simulink model "LKAS_AutoSave_DF_20220414_1924_SW62"  (R2018b)
settings: Solver=FixedStepDiscrete  StartTime=0.0  StopTime=10.0  FixedStep=0.01  RelTol=1e-3
model workspace (MAT data in the model file):
  MCOS : class17 (value not decoded)
  MCOS : class17 (value not decoded)
  MCOS : class17 (value not decoded)
  MCOS : class17 (value not decoded)
  MCOS : class17 (value not decoded)
  MCOS : class17 (value not decoded)
  MCOS : class17 (value not decoded)
  MCOS : class17 (value not decoded)
  MCOS : class17 (value not decoded)
  MCOS : class17 (value not decoded)
  MCOS : class17 (value not decoded)
  MCOS : class17 (value not decoded)
  MCOS : class17 (value not decoded)
  MCOS : class17 (value not decoded)
  MCOS : class17 (value not decoded)
  MCOS : class17 (value not decoded)
  MCOS : class17 (value not decoded)
  MCOS : class17 (value not decoded)
  MCOS : class17 (value not decoded)
  MCOS : class17 (value not decoded)
  MCOS : class17 (value not decoded)
  MCOS : class17 (value not decoded)
  MCOS : class17 (value not decoded)
  MCOS : class17 (value not decoded)
  MCOS : class17 (value not decoded)
  MCOS : class17 (value not decoded)
  MCOS : class17 (value not decoded)
  MCOS : class17 (value not decoded)
  MCOS : class17 (value not decoded)
  MCOS : class17 (value not decoded)
  MCOS : class17 (value not decoded)
  MCOS : class17 (value not decoded)
  MCOS : class17 (value not decoded)
  MCOS : class17 (value not decoded)
  MCOS : class17 (value not decoded)
  MCOS : class17 (value not decoded)
  MCOS : class17 (value not decoded)
  MCOS : class17 (value not decoded)
  MCOS : class17 (value not decoded)
  MCOS : class17 (value not decoded)
  MCOS : class17 (value not decoded)
  MCOS : class17 (value not decoded)
  MCOS : class17 (value not decoded)
  MCOS : class17 (value not decoded)
  MCOS : class17 (value not decoded)
  MCOS : class17 (value not decoded)
  MCOS : class17 (value not decoded)
  MCOS : class17 (value not decoded)
  MCOS : class17 (value not decoded)
  MCOS : class17 (value not decoded)
  MCOS : class17 (value not decoded)
  MCOS : class17 (value not decoded)
  MCOS : class17 (value not decoded)
  MCOS : class17 (value not decoded)
  MCOS : class17 (value not decoded)
  MCOS : class17 (value not decoded)
  MCOS : class17 (value not decoded)
  MCOS : class17 (value not decoded)
  MCOS : class17 (value not decoded)
  MCOS : class17 (value not decoded)
  MCOS : class17 (value not decoded)
  MCOS : class17 (value not decoded)
  MCOS : class17 (value not decoded)
  MCOS : class17 (value not decoded)
  MCOS : class17 (value not decoded)
  MCOS : class17 (value not decoded)
  MCOS : class17 (value not decoded)
  MCOS : class17 (value not decoded)
  MCOS : class17 (value not decoded)
  MCOS : class17 (value not decoded)
  MCOS : class17 (value not decoded)
  MCOS : class17 (value not decoded)
  MCOS : class17 (value not decoded)
  MCOS : class17 (value not decoded)
  MCOS : class17 (value not decoded)
  MCOS : class17 (value not decoded)
  MCOS : class17 (value not decoded)
  MCOS : class17 (value not decoded)
  MCOS : class17 (value not decoded)
  MCOS : class17 (value not decoded)
  MCOS : class17 (value not decoded)
  MCOS : class17 (value not decoded)
  MCOS : class17 (value not decoded)
  MCOS : class17 (value not decoded)
  MCOS : class17 (value not decoded)
  MCOS : class17 (value not decoded)
  MCOS : class17 (value not decoded)
  MCOS : class17 (value not decoded)
  MCOS : class17 (value not decoded)
  MCOS : class17 (value not decoded)
  MCOS : class17 (value not decoded)
  MCOS : class17 (value not decoded)
  MCOS : class17 (value not decoded)
  MCOS : class17 (value not decoded)
  MCOS : class17 (value not decoded)
  MCOS : class17 (value not decoded)
  MCOS : class17 (value not decoded)
  MCOS : class17 (value not decoded)
  MCOS : class17 (value not decoded)
  MCOS : class17 (value not decoded)
  MCOS : class17 (value not decoded)
  MCOS : class17 (value not decoded)
  MCOS : class17 (value not decoded)
  MCOS : class17 (value not decoded)
  MCOS : class17 (value not decoded)
  MCOS : class17 (value not decoded)
  MCOS : class17 (value not decoded)
  MCOS : class17 (value not decoded)
  MCOS : class17 (value not decoded)
undefined symbols (not defined in the file): LKA_CarWidth, LKA_SampleTime, LKA_StrRatio_C, LKA_Veh2CamL_C, LKA_Veh2CamW_C, LKA_WhlBaseL_C, LL_CompHdAg_C, LL_CompSWA_C, LL_CrvtPrvwT_C, LL_DesDvt_C, LL_DvtComp_C, LL_DvtPrvwT_C, LL_DvtSpdDet_vDvtSpdMin_C, LL_HandsOff_ExitTime, LL_HandsOff_TextTime, LL_HandsOff_WarnTime, LL_HdAgExT_C, LL_HdAgPrvwT_C, LL_LAccMax_C, LL_LAccRMax_C, LL_LDW_EarliestWarnLine_C, LL_LDW_LatestWarnLine_C, LL_LDWS_SUPPRESS_HEADING, LL_LFClb_TFC_FfCtlRatio_C, LL_LFClb_TFC_KdBalance_C, LL_LFClb_TFC_KdMaxSWA_C, LL_LFClb_TFC_KdV1_C, LL_LFClb_TFC_KdV2_C, LL_LFClb_TFC_KdVehSpdLwr_C, LL_LFClb_TFC_KdVehSpdUpr_C, LL_LFClb_TFC_Ki_C, LL_LFClb_TFC_KiMaxSWA_C, LL_LFClb_TFC_Kp_C, LL_LFClb_TFC_KpKlat_C, LL_LFClb_TFC_KpV1_C, LL_LFClb_TFC_KpV2_C, LL_LFClb_TFC_KpVehSpdLwr_C, LL_LFClb_TFC_KpVehSpdUpr_C, LL_LFClb_TFC_PrvwT_C, LL_LKA_EarliestWarnLine_C, LL_LKA_EnableLine_DvtMax, LL_LKA_EnableLine_DvtMin, LL_LKA_EnableLine_Max, LL_LKA_LatestWarnLine_C, LL_LKAExPrcs_ExitC0Dvt, LL_LKAExPrcs_ExitC0Swt, LL_LKAExPrcs_tiExitDelayTime3, LL_LKAExPrcs_tiExitTime1, LL_LKAExPrcs_tiExitTime2, LL_LKAExPrcs_tiExitTime3, LL_LKAS_OUT_OF_CONTROL_LAT_VEL, LL_LKAS_OUT_OF_CONTROL_TTLC, LL_LKASWASyn_M0, LL_LKASWASyn_M1, LL_LKASWASyn_M2, LL_LKASWASyn_M3D, LL_LKASWASyn_M3K_DT, LL_LKASWASyn_M3K_MSD, LL_LKASWASyn_M4K, LL_LKASWASyn_SWAaddMax ... (+50)
libraries: simulink x234, canmsglib x6, dspstat3 x3, simulink_extras x1
(part 4 of 17)

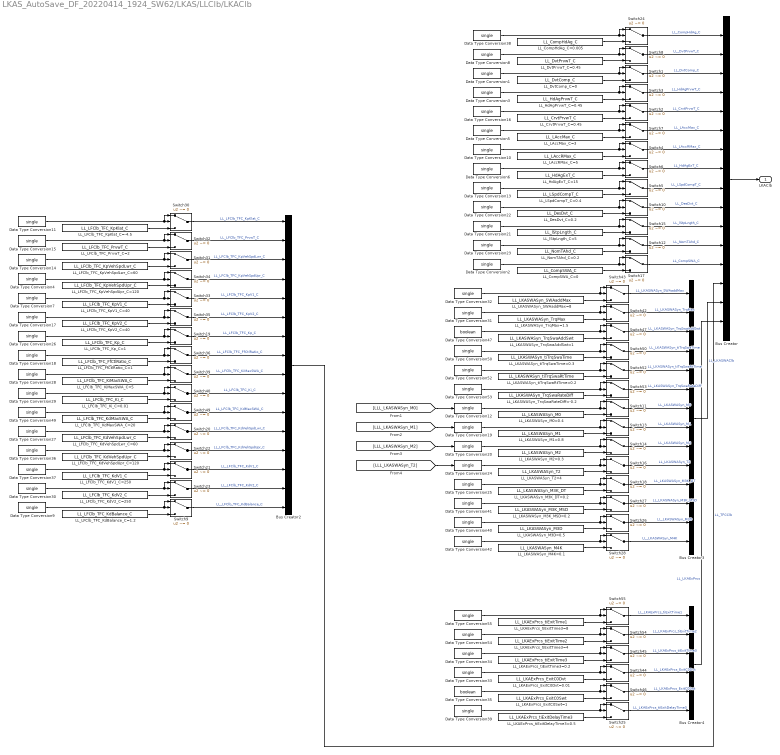
== system LKAS_AutoSave_DF_20220414_1924_SW62/LKAS/LLClb/LKAClb ==
  Bus Creator : BusCreator  Inputs=16
  Bus Creator2 : BusCreator  Inputs=16
  Bus Creator3 : BusCreator  Inputs=14
  Bus Creator4 : BusCreator  Inputs=6
  Data Type Conversion{1..34,36..42,49..50,52..55} (47 alike) : DataTypeConversion  OutDataTypeStr=single
  Data Type Conversion35 : DataTypeConversion  OutDataTypeStr=boolean
  Data Type Conversion47 : DataTypeConversion  OutDataTypeStr=boolean
  LL_CompHdAg_C=0.005 : Constant  Value=LL_CompHdAg_C  OutDataTypeStr=single
  LL_CompSWA_C=0 : Constant  Value=LL_CompSWA_C  OutDataTypeStr=single
  LL_CrvtPrvwT_C=0.45 : Constant  Value=LL_CrvtPrvwT_C  OutDataTypeStr=single
  LL_DesDvt_C=0.2 : Constant  Value=LL_DesDvt_C  OutDataTypeStr=single
  LL_DvtComp_C=0 : Constant  Value=LL_DvtComp_C  OutDataTypeStr=single
  LL_DvtPrvwT_C=0.45 : Constant  Value=LL_DvtPrvwT_C  OutDataTypeStr=single
  LL_HdAgExT_C=15 : Constant  Value=LL_HdAgExT_C  OutDataTypeStr=single
  LL_HdAgPrvwT_C=0.45 : Constant  Value=LL_HdAgPrvwT_C  OutDataTypeStr=single
  LL_LAccMax_C=3 : Constant  Value=LL_LAccMax_C  OutDataTypeStr=single
  LL_LAccRMax_C=5 : Constant  Value=LL_LAccRMax_C  OutDataTypeStr=single
  LL_LFClb_TFC_FfCtlRatio_C=1 : Constant  Value=LL_LFClb_TFC_FfCtlRatio_C  OutDataTypeStr=single
  LL_LFClb_TFC_KdBalance_C=1.2 : Constant  Value=LL_LFClb_TFC_KdBalance_C  OutDataTypeStr=single
  LL_LFClb_TFC_KdMaxSWA_C=20 : Constant  Value=LL_LFClb_TFC_KdMaxSWA_C  OutDataTypeStr=single
  LL_LFClb_TFC_KdV1_C=250 : Constant  Value=LL_LFClb_TFC_KdV1_C  OutDataTypeStr=single
  LL_LFClb_TFC_KdV2_C=250 : Constant  Value=LL_LFClb_TFC_KdV2_C  OutDataTypeStr=single
  LL_LFClb_TFC_KdVehSpdLwr_C=60 : Constant  Value=LL_LFClb_TFC_KdVehSpdLwr_C  OutDataTypeStr=single
  LL_LFClb_TFC_KdVehSpdUpr_C=120 : Constant  Value=LL_LFClb_TFC_KdVehSpdUpr_C  OutDataTypeStr=single
  LL_LFClb_TFC_KiMaxSWA_C=5 : Constant  Value=LL_LFClb_TFC_KiMaxSWA_C  OutDataTypeStr=single
  LL_LFClb_TFC_Ki_C=0.01 : Constant  Value=LL_LFClb_TFC_Ki_C  OutDataTypeStr=single
  LL_LFClb_TFC_KpKlat_C=-4.5 : Constant  Value=LL_LFClb_TFC_KpKlat_C  OutDataTypeStr=single
  LL_LFClb_TFC_KpV1_C=40 : Constant  Value=LL_LFClb_TFC_KpV1_C  OutDataTypeStr=single
  LL_LFClb_TFC_KpV2_C=40 : Constant  Value=LL_LFClb_TFC_KpV2_C  OutDataTypeStr=single
  LL_LFClb_TFC_KpVehSpdLwr_C=60 : Constant  Value=LL_LFClb_TFC_KpVehSpdLwr_C  OutDataTypeStr=single
  LL_LFClb_TFC_KpVehSpdUpr_C=120 : Constant  Value=LL_LFClb_TFC_KpVehSpdUpr_C  OutDataTypeStr=single
  LL_LFClb_TFC_Kp_C=1 : Constant  Value=LL_LFClb_TFC_Kp_C  OutDataTypeStr=single
  LL_LFClb_TFC_PrvwT_C=2 : Constant  Value=LL_LFClb_TFC_PrvwT_C  OutDataTypeStr=single
  LL_LKAExPrcs_ExitC0Dvt=0.01 : Constant  Value=LL_LKAExPrcs_ExitC0Dvt  OutDataTypeStr=single
  LL_LKAExPrcs_ExitC0Swt=1 : Constant  Value=LL_LKAExPrcs_ExitC0Swt  OutDataTypeStr=boolean
  LL_LKAExPrcs_tiExitDelayTime3=0.5 : Constant  Value=LL_LKAExPrcs_tiExitDelayTime3  OutDataTypeStr=single
  LL_LKAExPrcs_tiExitTime3=0.2 : Constant  Value=LL_LKAExPrcs_tiExitTime3  OutDataTypeStr=single
  LL_LKAExPrcs_tiExitTime3=4 : Constant  Value=LL_LKAExPrcs_tiExitTime2  OutDataTypeStr=single
  LL_LKAExPrcs_tiExitTime3=8 : Constant  Value=LL_LKAExPrcs_tiExitTime1  OutDataTypeStr=single
  LL_LKASWASyn_M0=0.4 : Constant  Value=LL_LKASWASyn_M0  OutDataTypeStr=single
  LL_LKASWASyn_M1=0.8 : Constant  Value=LL_LKASWASyn_M1  OutDataTypeStr=single
  LL_LKASWASyn_M2=0.3 : Constant  Value=LL_LKASWASyn_M2  OutDataTypeStr=single
  LL_LKASWASyn_M3D=0.5 : Constant  Value=LL_LKASWASyn_M3D  OutDataTypeStr=single
  LL_LKASWASyn_M3K_DT=0.2 : Constant  Value=LL_LKASWASyn_M3K_DT  OutDataTypeStr=single
  LL_LKASWASyn_M3K_MSD=0.2 : Constant  Value=LL_LKASWASyn_M3K_MSD  OutDataTypeStr=single
  LL_LKASWASyn_M4K=0.1 : Constant  Value=LL_LKASWASyn_M4K  OutDataTypeStr=single
  LL_LKASWASyn_SWAaddMax=8 : Constant  Value=LL_LKASWASyn_SWAaddMax  OutDataTypeStr=single
  LL_LKASWASyn_T2=4 : Constant  Value=LL_LKASWASyn_T2  OutDataTypeStr=single
  LL_LKASWASyn_TrqMax=1.5 : Constant  Value=LL_LKASWASyn_TrqMax  OutDataTypeStr=single
  LL_LKASWASyn_TrqSwaAddSwt=1 : Constant  Value=LL_LKASWASyn_TrqSwaAddSwt  OutDataTypeStr=boolean
  LL_LKASWASyn_TrqSwaRateDiff=-0.2 : Constant  Value=LL_LKASWASyn_TrqSwaRateDiff  OutDataTypeStr=single
  LL_LKASWASyn_tiTrqSwaRtTime=0.2 : Constant  Value=LL_LKASWASyn_tiTrqSwaRtTime  OutDataTypeStr=single
  LL_LKASWASyn_tiTrqSwaTime=0.3 : Constant  Value=LL_LKASWASyn_tiTrqSwaTime  OutDataTypeStr=single
  LL_LSpdCompT_C=0.4 : Constant  Value=LL_LSpdCompT_C  OutDataTypeStr=single
  LL_NomTAhd_C=0.2 : Constant  Value=LL_NomTAhd_C  OutDataTypeStr=single
  LL_lStpLngth_C=5 : Constant  Value=LL_lStpLngth_C  OutDataTypeStr=single
  Switch{1..28,30..36,39..40,42..45,49..50,52..55} (47 alike) : Switch  Criteria=u2 ~= 0  OutDataTypeStr=single
  Switch46 : Switch  Criteria=u2 ~= 0  OutDataTypeStr=boolean
  Switch47 : Switch  Criteria=u2 ~= 0  OutDataTypeStr=boolean
  LKAClb : Outport
  wires:
  Data Type Conversion42/1 -> Switch28/2, Switch28/1
  LL_LKASWASyn_M4K=0.1/1 -> Switch28/3
  Switch28/1 -> Bus Creator3/14  "LL_LKASWASyn_M4K"
  Switch27/1 -> Bus Creator3/12  "LL_LKASWASyn_M3K_MSD"
  LL_LKASWASyn_M3K_MSD=0.2/1 -> Switch27/3
  Data Type Conversion41/1 -> Switch27/1, Switch27/2
  Switch26/1 -> Bus Creator3/13  "LL_LKASWASyn_M3D"
  LL_LKASWASyn_M3D=0.5/1 -> Switch26/3
  Data Type Conversion40/1 -> Switch26/1, Switch26/2
  Data Type Conversion39/1 -> Switch25/2, Switch25/1
  Switch25/1 -> Bus Creator4/6  "LL_LKAExPrcs_tiExitDelayTime3"
  LL_LKAExPrcs_tiExitDelayTime3=0.5/1 -> Switch25/3
  LL_CompHdAg_C=0.005/1 -> Switch24/3
  Data Type Conversion38/1 -> Switch24/1, Switch24/2
  Switch24/1 -> Bus Creator/1  "LL_CompHdAg_C"
  Data Type Conversion37/1 -> Switch21/2, Switch21/1
  LL_LFClb_TFC_KdV2_C=250/1 -> Switch23/3
  Switch23/1 -> Bus Creator2/15  "LL_LFClb_TFC_KdV2_C"
  LL_LFClb_TFC_KdVehSpdUpr_C=120/1 -> Switch22/3
  Switch20/1 -> Bus Creator2/12  "LL_LFClb_TFC_KdVehSpdLwr_C"
  Switch22/1 -> Bus Creator2/13  "LL_LFClb_TFC_KdVehSpdUpr_C"
  Data Type Conversion27/1 -> Switch20/2, Switch20/1
  Data Type Conversion36/1 -> Switch22/2, Switch22/1
  LL_LFClb_TFC_KdV1_C=250/1 -> Switch21/3
  LL_LFClb_TFC_KdVehSpdLwr_C=60/1 -> Switch20/3
  Switch21/1 -> Bus Creator2/14  "LL_LFClb_TFC_KdV1_C"
  Data Type Conversion30/1 -> Switch23/2, Switch23/1
  LL_LFClb_TFC_Kp_C=1/1 -> Switch19/3
  Switch19/1 -> Bus Creator2/7  "LL_LFClb_TFC_Kp_C"
  Data Type Conversion26/1 -> Switch19/2, Switch19/1
  Bus Creator/1 -> LKAClb/1
  Switch8/1 -> Bus Creator/2  "LL_DvtPrvwT_C"
  Switch1/1 -> Bus Creator/3  "LL_DvtComp_C"
  Switch3/1 -> Bus Creator/4  "LL_HdAgPrvwT_C"
  Switch17/1 -> Bus Creator/13  "LL_CompSWA_C"
  Switch6/1 -> Bus Creator/8  "LL_HdAgExT_C"
  Switch7/1 -> Bus Creator/6  "LL_LAccMax_C"
  Switch4/1 -> Bus Creator/7  "LL_LAccRMax_C"
  Switch5/1 -> Bus Creator/9  "LL_LSpdCompT_C"
  Switch2/1 -> Bus Creator/5  "LL_CrvtPrvwT_C"
  Switch15/1 -> Bus Creator/11  "LL_lStpLngth_C"
  Switch10/1 -> Bus Creator/10  "LL_DesDvt_C"
  Switch12/1 -> Bus Creator/12  "LL_NomTAhd_C"
  LL_DvtPrvwT_C=0.45/1 -> Switch8/3
  Data Type Conversion8/1 -> Switch8/1, Switch8/2
  Data Type Conversion1/1 -> Switch1/2, Switch1/1
  LL_DvtComp_C=0/1 -> Switch1/3
  LL_CrvtPrvwT_C=0.45/1 -> Switch2/3
  Data Type Conversion16/1 -> Switch2/2, Switch2/1
  Data Type Conversion3/1 -> Switch3/2, Switch3/1
  LL_HdAgPrvwT_C=0.45/1 -> Switch3/3
  LL_HdAgExT_C=15/1 -> Switch6/3
  Data Type Conversion6/1 -> Switch6/2, Switch6/1
  Data Type Conversion13/1 -> Switch5/2, Switch5/1
  LL_LSpdCompT_C=0.4/1 -> Switch5/3
  LL_LAccRMax_C=5/1 -> Switch4/3
  Data Type Conversion10/1 -> Switch4/1, Switch4/2
  Data Type Conversion5/1 -> Switch7/2, Switch7/1
  LL_LAccMax_C=3/1 -> Switch7/3
  Data Type Conversion21/1 -> Switch15/2, Switch15/1
  Data Type Conversion23/1 -> Switch12/2, Switch12/1
  Data Type Conversion22/1 -> Switch10/2, Switch10/1
  Data Type Conversion2/1 -> Switch17/2, Switch17/1
  LL_DesDvt_C=0.2/1 -> Switch10/3
  LL_lStpLngth_C=5/1 -> Switch15/3
  LL_NomTAhd_C=0.2/1 -> Switch12/3
  LL_CompSWA_C=0/1 -> Switch17/3
  Bus Creator2/1 -> Bus Creator/14  "LL_TFCClb"
  Switch35/1 -> Bus Creator2/6  "LL_LFClb_TFC_KpV2_C"
  Switch30/1 -> Bus Creator2/1  "LL_LFClb_TFC_KpKlat_C"
  Switch31/1 -> Bus Creator2/3  "LL_LFClb_TFC_KpVehSpdLwr_C"
  Switch34/1 -> Bus Creator2/4  "LL_LFClb_TFC_KpVehSpdUpr_C"
  Switch33/1 -> Bus Creator2/5  "LL_LFClb_TFC_KpV1_C"
  Switch32/1 -> Bus Creator2/2  "LL_LFClb_TFC_PrvwT_C"
  LL_LFClb_TFC_KpV1_C=40/1 -> Switch33/3
  LL_LFClb_TFC_KpVehSpdLwr_C=60/1 -> Switch31/3
  LL_LFClb_TFC_PrvwT_C=2/1 -> Switch32/3
  Data Type Conversion11/1 -> Switch30/2, Switch30/1
  Data Type Conversion7/1 -> Switch33/2, Switch33/1
  Data Type Conversion4/1 -> Switch34/2, Switch34/1
  Data Type Conversion15/1 -> Switch32/2, Switch32/1
  Data Type Conversion17/1 -> Switch35/2, Switch35/1
  LL_LFClb_TFC_KpV2_C=40/1 -> Switch35/3
  Data Type Conversion14/1 -> Switch31/2, Switch31/1
  LL_LFClb_TFC_KpVehSpdUpr_C=120/1 -> Switch34/3
  LL_LFClb_TFC_KpKlat_C=-4.5/1 -> Switch30/3
  LL_LFClb_TFC_FfCtlRatio_C=1/1 -> Switch36/3
  Data Type Conversion18/1 -> Switch36/1, Switch36/2
  Switch36/1 -> Bus Creator2/8  "LL_LFClb_TFC_FfCtlRatio_C"
  Switch40/1 -> Bus Creator2/10  "LL_LFClb_TFC_Ki_C"
  Switch39/1 -> Bus Creator2/9  "LL_LFClb_TFC_KiMaxSWA_C"
  LL_LFClb_TFC_KiMaxSWA_C=5/1 -> Switch39/3
  Data Type Conversion28/1 -> Switch39/1, Switch39/2
  LL_LFClb_TFC_Ki_C=0.01/1 -> Switch40/3
  Data Type Conversion29/1 -> Switch40/1, Switch40/2
  Data Type Conversion31/1 -> Switch42/2, Switch42/1
  LL_LKASWASyn_TrqMax=1.5/1 -> Switch42/3
  LL_LKASWASyn_SWAaddMax=8/1 -> Switch43/3
  Data Type Conversion32/1 -> Switch43/1, Switch43/2
  Switch43/1 -> Bus Creator3/1  "LL_LKASWASyn_SWAaddMax"
  Switch42/1 -> Bus Creator3/2  "LL_LKASWASyn_TrqMax"
  Bus Creator3/1 -> Bus Creator/15  "LL_LKASWAClb"
  Switch44/1 -> Bus Creator4/4  "LL_LKAExPrcs_ExitC0Dvt"
  Switch45/1 -> Bus Creator4/3  "LL_LKAExPrcs_tiExitTime3"
  Data Type Conversion34/1 -> Switch45/2, Switch45/1
  LL_LKAExPrcs_tiExitTime3=0.2/1 -> Switch45/3
  LL_LKAExPrcs_ExitC0Dvt=0.01/1 -> Switch44/3
  Data Type Conversion33/1 -> Switch44/1, Switch44/2
  Bus Creator4/1 -> Bus Creator/16  "LL_LKAExPrcs"
  Data Type Conversion35/1 -> Switch46/2, Switch46/1
  LL_LKAExPrcs_ExitC0Swt=1/1 -> Switch46/3
  Switch46/1 -> Bus Creator4/5  "LL_LKAExPrcs_ExitC0Swt"
  Switch47/1 -> Bus Creator3/3  "LL_LKASWASyn_TrqSwaAddSwt"
  LL_LKASWASyn_TrqSwaAddSwt=1/1 -> Switch47/3
  Data Type Conversion47/1 -> Switch47/1, Switch47/2
  Switch49/1 -> Bus Creator2/11  "LL_LFClb_TFC_KdMaxSWA_C"
  LL_LFClb_TFC_KdMaxSWA_C=20/1 -> Switch49/3
  Data Type Conversion49/1 -> Switch49/1, Switch49/2
  Data Type Conversion50/1 -> Switch50/2, Switch50/1
  LL_LKASWASyn_tiTrqSwaTime=0.3/1 -> Switch50/3
  Switch50/1 -> Bus Creator3/4  "LL_LKASWASyn_tiTrqSwaTime"
  Switch52/1 -> Bus Creator3/5  "LL_LKASWASyn_tiTrqSwaRtTime"
  LL_LKASWASyn_tiTrqSwaRtTime=0.2/1 -> Switch52/3
  Data Type Conversion52/1 -> Switch52/1, Switch52/2
  Data Type Conversion53/1 -> Switch53/2, Switch53/1
  LL_LKASWASyn_TrqSwaRateDiff=-0.2/1 -> Switch53/3
  Switch53/1 -> Bus Creator3/6  "LL_LKASWASyn_TrqSwaRateDiff"
  LL_LKAExPrcs_tiExitTime3=4/1 -> Switch54/3
  Data Type Conversion54/1 -> Switch54/1, Switch54/2
  Switch54/1 -> Bus Creator4/2  "LL_LKAExPrcs_tiExitTime2"
  Switch55/1 -> Bus Creator4/1  "LL_LKAExPrcs_tiExitTime1"
  Data Type Conversion55/1 -> Switch55/2, Switch55/1
  LL_LKAExPrcs_tiExitTime3=8/1 -> Switch55/3
  Switch9/1 -> Bus Creator2/16  "LL_LFClb_TFC_KdBalance_C"
  LL_LFClb_TFC_KdBalance_C=1.2/1 -> Switch9/3
  Data Type Conversion9/1 -> Switch9/1, Switch9/2
  [LLL_LKASWASyn_T2] -> Data Type Conversion24/1
  Switch16/1 -> Bus Creator3/10  "LL_LKASWASyn_T2"
  LL_LKASWASyn_T2=4/1 -> Switch16/3
  Data Type Conversion24/1 -> Switch16/1, Switch16/2
  Data Type Conversion20/1 -> Switch14/2, Switch14/1
  LL_LKASWASyn_M2=0.3/1 -> Switch14/3
  Switch14/1 -> Bus Creator3/9  "LL_LKASWASyn_M2"
  [LLL_LKASWASyn_M2] -> Data Type Conversion20/1
  [LLL_LKASWASyn_M1] -> Data Type Conversion19/1
  Switch13/1 -> Bus Creator3/8  "LL_LKASWASyn_M1"
  LL_LKASWASyn_M1=0.8/1 -> Switch13/3
  Data Type Conversion19/1 -> Switch13/1, Switch13/2
  Data Type Conversion12/1 -> Switch11/2, Switch11/1
  LL_LKASWASyn_M0=0.4/1 -> Switch11/3
  Switch11/1 -> Bus Creator3/7  "LL_LKASWASyn_M0"
  [LLL_LKASWASyn_M0] -> Data Type Conversion12/1
  Data Type Conversion25/1 -> Switch18/2, Switch18/1
  LL_LKASWASyn_M3K_DT=0.2/1 -> Switch18/3
  Switch18/1 -> Bus Creator3/11  "LL_LKASWASyn_M3K_DT"

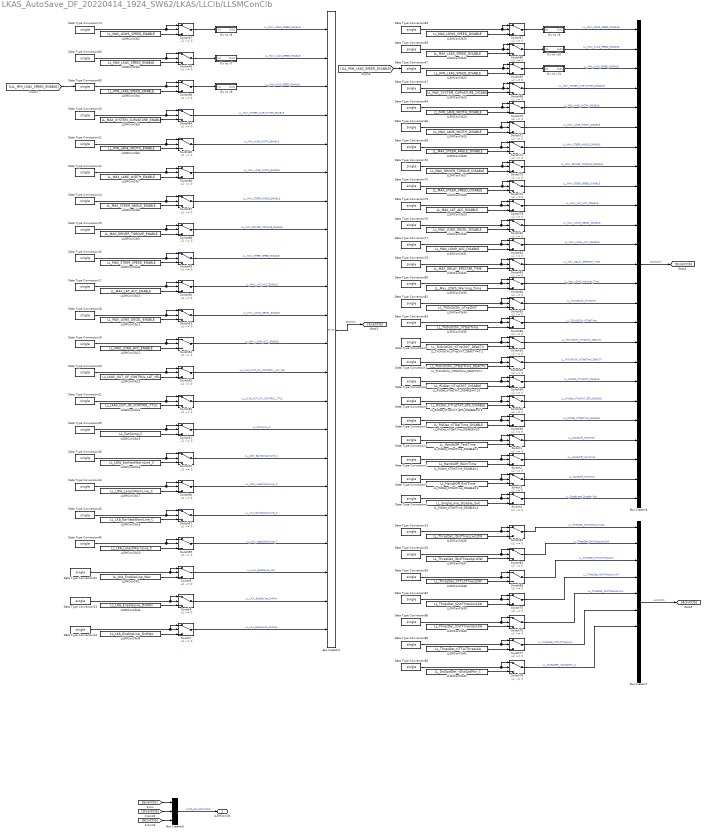
== system LKAS_AutoSave_DF_20220414_1924_SW62/LKAS/LLClb/LLSMConClb ==
  Bus Creator4 : BusCreator  Inputs=22
  Bus Creator5 : BusCreator  Inputs=3
  Bus Creator6 : BusCreator  Inputs=25
  Bus Creator7 : BusCreator  Inputs=10
  Data Type Conversion{1..26,36,44..47,58,64..70,72,74..78,80,82..89} (54 alike) : DataTypeConversion  OutDataTypeStr=single
  ICv to v10 : Subsystem
  ICv to v11 : Subsystem
  ICv to v6 : Subsystem  Description=|
      | 仪表车速转换
      | 仪表车速 = 实际车速 * 1.02 + 2.5
      settings: AttributesFormatString=%<Description>
  ICv to v7 : Subsystem
  ICv to v8 : Subsystem
  ICv to v9 : Subsystem
  LLSMConClb1 : Constant  Description=LKA功能的偏移量使能上限  Value=LL_LKA_EnableLine_Max  OutDataTypeStr=single
      settings: AttributesFormatString=|
      | %<Value>  = 0.4
      | %<Description>
  LLSMConClb10 : Constant  Description=侧向加速度使能上限  Value=LL_MAX_LAT_ACC_ENABLE  OutDataTypeStr=single
      settings: AttributesFormatString=|
      | %<Value>  = 3
      | %<Description>
  LLSMConClb11 : Constant  Description=纵向减速度使能上限  Value=LL_MAX_LONG_DECEL_ENABLE  OutDataTypeStr=single
      settings: AttributesFormatString=|
      | %<Value>  = 2
      | %<Description>
  LLSMConClb12 : Constant  Description=纵向加速度使能上限  Value=LL_MAX_LONG_ACC_ENABLE  OutDataTypeStr=single
      settings: AttributesFormatString=|
      | %<Value>  = 3
      | %<Description>
  LLSMConClb13 : Constant  Description=LKA功能的侧向偏出速度阈值  Value=LL_LKAS_OUT_OF_CONTROL_LAT_VEL  OutDataTypeStr=single
      settings: AttributesFormatString=|
      | %<Value>  = 1.5
      | %<Description>
  LLSMConClb14 : Constant  Description=LKA功能的超过最迟干预线持续时间阈值  Value=LL_LKAS_OUT_OF_CONTROL_TTLC  OutDataTypeStr=single
      settings: AttributesFormatString=|
      | %<Value>  = 0.3
      | %<Description>
  LLSMConClb15 : Constant  Description=偏移量补偿  Value=LL_DvtComp_C  OutDataTypeStr=single
      settings: AttributesFormatString=|
      | %<Value>  = 0
      | %<Description>
  LLSMConClb16 : Constant  Description=LDW功能的最早预警线  Value=LL_LDW_EarliestWarnLine_C  OutDataTypeStr=single
      settings: AttributesFormatString=|
      | %<Value>  = 0.3
      | %<Description>
  LLSMConClb17 : Constant  Description=LDW功能的最迟预警线  Value=LL_LDW_LatestWarnLine_C  OutDataTypeStr=single
      settings: AttributesFormatString=|
      | %<Value>  = -0.4
      | %<Description>
  LLSMConClb18 : Constant  Description=LKA功能的最早预警线  Value=LL_LKA_EarliestWarnLine_C  OutDataTypeStr=single
      settings: AttributesFormatString=|
      | %<Value>  = 0.3
      | %<Description>
  LLSMConClb19 : Constant  Description=LKA功能的最迟预警线  Value=LL_LKA_LatestWarnLine_C  OutDataTypeStr=single
      settings: AttributesFormatString=|
      | %<Value>  = -0.5
      | %<Description>
  LLSMConClb2 : Constant  Description=LDW功能的车速使能上限  Value=LL_MAX_LDWS_SPEED_ENABLE  OutDataTypeStr=single
      settings: AttributesFormatString=|
      | %<Value>  = 140
      | %<Description>
  LLSMConClb20 : Constant  Description=LDW功能的车速失效上限  Value=LL_MAX_LDWS_SPEED_DISABLE  OutDataTypeStr=single
      settings: AttributesFormatString=|
      | %<Value>  = 150
      | %<Description>
  LLSMConClb21 : Constant  Description=LKA功能的车速失效上限  Value=LL_MAX_LKAS_SPEED_DISABLE  OutDataTypeStr=single
      settings: AttributesFormatString=|
      | %<Value>  = 150
      | %<Description>
  LLSMConClb22 : Constant  Description=LKA功能的车速失效下限  Value=LL_MIN_LKAS_SPEED_DISABLE  OutDataTypeStr=single
      settings: AttributesFormatString=|
      | %<Value>  = 55
      | %<Description>
  LLSMConClb23 : Constant  Description=曲率失效上限  Value=LL_MAX_SYSTEM_CURVATURE_DISABLE  OutDataTypeStr=single
      settings: AttributesFormatString=|
      | %<Value>  = 0.0055
      | %<Description>
  LLSMConClb24 : Constant  Description=车道线宽度失效下限  Value=LL_MIN_LANE_WIDTH_DISABLE  OutDataTypeStr=single
      settings: AttributesFormatString=|
      | %<Value>  = 2.4
      | %<Description>
  LLSMConClb25 : Constant  Description=车道线宽度失效上限  Value=LL_MAX_LANE_WIDTH_DISABLE  OutDataTypeStr=single
      settings: AttributesFormatString=|
      | %<Value>  = 5.5
      | %<Description>
  LLSMConClb26 : Constant  Description=方向盘转角退出上限  Value=LL_MAX_STEER_ANGLE_DISABLE  OutDataTypeStr=single
      settings: AttributesFormatString=|
      | %<Value>  = 70
      | %<Description>
  LLSMConClb27 : Constant  Description=驾驶员转矩失效上限  Value=LL_MAX_DRIVER_TORQUE_DISABLE  OutDataTypeStr=single
      settings: AttributesFormatString=|
      | %<Value>  = 2.25
      | %<Description>
  LLSMConClb28 : Constant  Description=方向盘转速失效上限  Value=LL_MAX_STEER_SPEED_DISABLE  OutDataTypeStr=single
      settings: AttributesFormatString=|
      | %<Value>  = 5000
      | %<Description>
  LLSMConClb29 : Constant  Description=侧向加速度失效上限  Value=LL_MAX_LAT_ACC_DISABLE  OutDataTypeStr=single
      settings: AttributesFormatString=|
      | %<Value>  = 3.5
      | %<Description>
  LLSMConClb3 : Constant  Description=LKA功能的车速使能上限  Value=LL_MAX_LKAS_SPEED_ENABLE  OutDataTypeStr=single
      settings: AttributesFormatString=|
      | %<Value>  = 140
      | %<Description>
  LLSMConClb30 : Constant  Description=纵向减速度失效上限  Value=LL_MAX_LONG_DECEL_DISABLE  OutDataTypeStr=single
      settings: AttributesFormatString=|
      | %<Value>  = 2.5
      | %<Description>
  LLSMConClb31 : Constant  Description=纵向加速度失效上限  Value=LL_MAX_LONG_ACC_DISABLE  OutDataTypeStr=single
      settings: AttributesFormatString=|
      | %<Value>  = 3.5
      | %<Description>
  LLSMConClb32 : Constant  Description=LKA功能的EPS延迟进入等待的时间上限  Value=LL_MAX_DELAY_EPSSTAR_TIME  OutDataTypeStr=single
      settings: AttributesFormatString=|
      | %<Value>  = 0.5
      | %<Description>
  LLSMConClb33 : Constant  Description=LDW功能的连续报警时间上限  Value=LL_Max_LDWS_Warning_Time  OutDataTypeStr=single
      settings: AttributesFormatString=|
      | %<Value>  = 5
      | %<Description>
  LLSMConClb34 : Constant  Description=驾驶员接管时间阈值  Value=LL_TkOvStChk_tiTrqChkT  OutDataTypeStr=single
      settings: AttributesFormatString=|
      | %<Value>  = 0.1
      | %<Description>
  LLSMConClb35 : Constant  Description=距离上次驾驶员接管时间间隔  Value=LL_TkOvStChk_tiTDelTime  OutDataTypeStr=single
      settings: AttributesFormatString=|
      | %<Value>  = 2
      | %<Description>
  LLSMConClb36 : Constant  Description=LDW功能的偏移量激活下限  Value=LL_ThresDet_lDvtThresLwrLDW  OutDataTypeStr=single
      settings: AttributesFormatString=|
      | %<Value>  = 0.15
      | %<Description>
  LLSMConClb37 : Constant  Description=LDW功能的偏移量激活上限  Value=LL_ThresDet_lDvtThresUprLDW  OutDataTypeStr=single
      settings: AttributesFormatString=|
      | %<Value>  = 0.3
      | %<Description>
  LLSMConClb38 : Constant  Description=LDW功能的跨道时间激活阈值  Value=LL_ThresDet_tiTTLCThresLDW  OutDataTypeStr=single
      settings: AttributesFormatString=|
      | %<Value>  = 0.75
      | %<Description>
  LLSMConClb39 : Constant  Description=LKA功能的偏移量激活下限  Value=LL_ThresDet_lDvtThresLwrLKA  OutDataTypeStr=single
      settings: AttributesFormatString=|
      | %<Value>  = 0.3
      | %<Description>
  LLSMConClb4 : Constant  Description=LKA功能的车速使能下限  Value=LL_MIN_LKAS_SPEED_ENABLE  OutDataTypeStr=single
      settings: AttributesFormatString=|
      | %<Value>  = 60
      | %<Description>
  LLSMConClb40 : Constant  Description=LKA功能的偏移量激活上限  Value=LL_ThresDet_lDvtThresUprLKA  OutDataTypeStr=single
      settings: AttributesFormatString=|
      | %<Value>  = 0.6
      | %<Description>
  LLSMConClb41 : Constant  Description=LKA功能的跨道时间激活阈值  Value=LL_ThresDet_tiTTLCThresLKA  OutDataTypeStr=single
      settings: AttributesFormatString=|
      | %<Value>  = 1.5
      | %<Description>
  LLSMConClb42 : Constant  Description=偏出侧向速度最小值  Value=LL_DvtSpdDet_vDvtSpdMin_C  OutDataTypeStr=single
      settings: AttributesFormatString=|
      | %<Value>  = 0
      | %<Description>
  LLSMConClb43 : Constant  Description=方向盘转速使能上限  Value=LL_MAX_STEER_SPEED_ENABLE  OutDataTypeStr=single
      settings: AttributesFormatString=|
      | %<Value>  = 5000
      | %<Description>
  LLSMConClb44 : Constant  Description=LKA功能的使能最小车道宽度计算因子  Value=LL_LKA_EnableLine_DvtMin  OutDataTypeStr=single
      settings: AttributesFormatString=|
      | %<Value>  = 0.2
      | %<Description>
  LLSMConClb45 : Constant  Description=LKA功能的使能最大车道宽度计算因子  Value=LL_LKA_EnableLine_DvtMax  OutDataTypeStr=single
      settings: AttributesFormatString=|
      | %<Value>  = 1.2
      | %<Description>
  LLSMConClb5 : Constant  Description=曲率使能上限  Value=LL_MAX_SYSTEM_CURVATURE_ENABLE  OutDataTypeStr=single
      settings: AttributesFormatString=|
      | %<Value>  = 0.0045
      | %<Description>
  LLSMConClb6 : Constant  Description=车道线宽度使能下限  Value=LL_MIN_LANE_WIDTH_ENABLE  OutDataTypeStr=single
      settings: AttributesFormatString=|
      | %<Value>  = 2.5
      | %<Description>
  LLSMConClb7 : Constant  Description=车道线宽度使能上限  Value=LL_MAX_LANE_WIDTH_ENABLE  OutDataTypeStr=single
      settings: AttributesFormatString=|
      | %<Value>  = 5.4
      | %<Description>
  LLSMConClb8 : Constant  Description=方向盘转角使能上限  Value=LL_MAX_STEER_ANGLE_ENABLE  OutDataTypeStr=single
      settings: AttributesFormatString=|
      | %<Value>  = 60
      | %<Description>
  LLSMConClb9 : Constant  Description=驾驶员扭矩使能上限  Value=LL_MAX_DRIVER_TORQUE_ENABLE  OutDataTypeStr=single
      settings: AttributesFormatString=|
      | %<Value>  = 3
      | %<Description>
  LL_RlsDet_tiTDelTime_DISABLE=1 : Constant  Description=驾驶员脱手开始到功能发出动画提醒的时间  Value=LL_HandsOff_TextTime  OutDataTypeStr=single
      settings: AttributesFormatString=|
      | %<Value>  = 10
      | %<Description>
  LL_RlsDet_tiTDelTime_DISABLE=2 : Constant  Description=驾驶员脱手开始到发出声音报警的时间  Value=LL_HandsOff_WarnTime  OutDataTypeStr=single
      settings: AttributesFormatString=|
      | %<Value>  = 15
      | %<Description>
  LL_RlsDet_tiTDelTime_DISABLE=20 : Constant  Description=反使能距离上次驾驶员脱手时间间隔  Value=LL_RlsDet_tiTDelTime_DISABLE  OutDataTypeStr=single
      settings: AttributesFormatString=|
      | %<Value>  = 20
      | %<Description>
  LL_RlsDet_tiTDelTime_DISABLE=3 : Constant  Description=驾驶员脱手开始到功能退出的时间  Value=LL_HandsOff_ExitTime  OutDataTypeStr=single
      settings: AttributesFormatString=|
      | %<Value>  = 20
      | %<Description>
  LL_RlsDet_tiTDelTime_DISABLE=4 : Constant  Description=驾驶员脱手开始到功能退出的时间  Value=LL_SingleLane_Disable_Swt  OutDataTypeStr=boolean
      settings: AttributesFormatString=|
      | %<Value>  = 0
      | %<Description>
  LL_RlsDet_tiTrqChkT_DISABLE=0.25 : Constant  Description=反使能驾驶员脱手时间阈值  Value=LL_RlsDet_tiTrqChkT_DISABLE  OutDataTypeStr=single
      settings: AttributesFormatString=|
      | %<Value>  = 0.25
      | %<Description>
  LL_RlsDet_tiTrqChkT_EPS_DISABLE=0.5 : Constant  Description=反使能驾驶员脱手时间阈值（EPS激活）  Value=LL_RlsDet_tiTrqChkT_EPS_DISABLE  OutDataTypeStr=single
      settings: AttributesFormatString=|
      | %<Value>  = 0.5
      | %<Description>
  LL_TkOvStChk_tiTDelTime_DEACTV=1 : Constant  Description=取消激活距离上次驾驶员接管时间间隔  Value=LL_TkOvStChk_tiTDelTime_DEACTV  OutDataTypeStr=single
      settings: AttributesFormatString=|
      | %<Value>  = 1
      | %<Description>
  LL_TkOvStChk_tiTrqChkT_DEACTV=0.2 : Constant  Description=取消激活驾驶员接管时间阈值  Value=LL_TkOvStChk_tiTrqChkT_DEACTV  OutDataTypeStr=single
      settings: AttributesFormatString=|
      | %<Value>  = 0.2
      | %<Description>
  Switch{1..3,5..7,16,38,40,44,46..88} (53 alike) : Switch  Criteria=u2 ~= 0  OutDataTypeStr=single
  Switch4 : Switch  Criteria=u2 ~= 0  OutDataTypeStr=boolean
  LLSMConClb : Outport
  wires:
  Switch4/1 -> Bus Creator6/25  "LL_SingleLane_Disable_Swt"
  LL_RlsDet_tiTDelTime_DISABLE=4/1 -> Switch4/3
  Data Type Conversion4/1 -> Switch4/1, Switch4/2
  Data Type Conversion3/1 -> Switch3/2, Switch3/1
  LL_RlsDet_tiTDelTime_DISABLE=3/1 -> Switch3/3
  Switch3/1 -> Bus Creator6/24  "LL_HandsOff_ExitTime"
  Switch2/1 -> Bus Creator6/23  "LL_HandsOff_WarnTime"
  LL_RlsDet_tiTDelTime_DISABLE=2/1 -> Switch2/3
  Data Type Conversion2/1 -> Switch2/1, Switch2/2
  Data Type Conversion1/1 -> Switch1/2, Switch1/1
  Switch1/1 -> Bus Creator6/22  "LL_HandsOff_TextTime"
  LL_RlsDet_tiTDelTime_DISABLE=1/1 -> Switch1/3
  LL_RlsDet_tiTrqChkT_EPS_DISABLE=0.5/1 -> Switch44/3
  Switch44/1 -> Bus Creator6/20  "LL_RlsDet_tiTrqChkT_EPS_DISABLE"
  Data Type Conversion6/1 -> Switch38/2, Switch38/1
  LL_TkOvStChk_tiTDelTime_DEACTV=1/1 -> Switch40/3
  LL_RlsDet_tiTDelTime_DISABLE=20/1 -> Switch46/3
  Switch46/1 -> Bus Creator6/21  "LL_RlsDet_tiTDelTime_DISABLE"
  Data Type Conversion8/1 -> Switch44/1, Switch44/2
  Data Type Conversion9/1 -> Switch46/1, Switch46/2
  Switch40/1 -> Bus Creator6/18  "LL_TkOvStChk_tiTDelTime_DEACTV"
  Switch16/1 -> Bus Creator6/17  "LL_TkOvStChk_tiTrqChkT_DEACTV"
  Data Type Conversion5/1 -> Switch16/2, Switch16/1
  Switch38/1 -> Bus Creator6/19  "LL_RlsDet_tiTrqChkT_DISABLE"
  Data Type Conversion7/1 -> Switch40/1, Switch40/2
  LL_TkOvStChk_tiTrqChkT_DEACTV=0.2/1 -> Switch16/3
  LL_RlsDet_tiTrqChkT_DISABLE=0.25/1 -> Switch38/3
  Data Type Conversion25/1 -> Switch51/2, Switch51/1
  LLSMConClb2/1 -> Switch47/3
  Switch56/1 -> Bus Creator4/14  "LL_LKAS_OUT_OF_CONTROL_TTLC"
  Data Type Conversion89/1 -> Switch58/2, Switch58/1
  Switch86/1 -> Bus Creator4/6  "LL_MAX_LANE_WIDTH_ENABLE"
  Switch88/1 -> Bus Creator4/8  "LL_MAX_DRIVER_TORQUE_ENABLE"
  Data Type Conversion74/1 -> Switch47/2, Switch47/1
  Data Type Conversion75/1 -> Switch79/1, Switch79/2
  LLSMConClb28/1 -> Switch74/3
  Data Type Conversion45/1 -> Switch57/2, Switch57/1
  [LLL_MIN_LKAS_SPEED_ENABLE] -> Data Type Conversion89/1
  LLSMConClb13/1 -> Switch55/3
  Switch68/1 -> Bus Creator6/4  "LL_MAX_SYSTEM_CURVATURE_DISABLE"
  LLSMConClb32/1 -> Switch63/3
  LLSMConClb15/1 -> Switch51/3
  Data Type Conversion80/1 -> Switch64/2, Switch64/1
  Data Type Conversion26/1 -> Switch82/1, Switch82/2
  Switch57/1 -> Bus Creator4/18  "LL_LKA_EarliestWarnLine_C"
  Data Type Conversion83/1 -> Switch66/2, Switch66/1
  Data Type Conversion12/1 -> Switch86/2, Switch86/1
  Data Type Conversion15/1 -> Switch88/2, Switch88/1
  Switch58/1 -> ICv to v8/1(In1)
  Data Type Conversion86/1 -> Switch78/1, Switch78/2
  Switch71/1 -> Bus Creator6/6  "LL_MAX_LANE_WIDTH_DISABLE"
  Bus Creator4/1 -> [EnaCClb]  "EnaCClb"
  Switch72/1 -> Bus Creator6/7  "LL_MAX_STEER_ANGLE_DISABLE"
  Switch62/1 -> Bus Creator6/12  "LL_MAX_LONG_ACC_DISABLE"
  LLSMConClb6/1 -> Switch85/3
  Switch60/1 -> Bus Creator4/17  "LL_LDW_LatestWarnLine_C"
  Data Type Conversion21/1 -> Switch56/2, Switch56/1
  Data Type Conversion47/1 -> Switch68/2, Switch68/1
  Switch87/1 -> Bus Creator4/7  "LL_MAX_STEER_ANGLE_ENABLE"
  LLSMConClb20/1 -> Switch67/3
  Switch47/1 -> ICv to v6/1(In1)
  LLSMConClb17/1 -> Switch60/3
  Switch54/1 -> Bus Creator4/12  "LL_MAX_LONG_ACC_ENABLE"
  LLSMConClb22/1 -> Switch69/3
  LLSMConClb36/1 -> Switch81/3
  Switch67/1 -> ICv to v9/1(In1)
  Data Type Conversion85/1 -> Switch77/2, Switch77/1
  LLSMConClb42/1 -> Switch78/3
  Data Type Conversion67/1 -> Switch69/1, Switch69/2
  Switch65/1 -> Bus Creator6/15  "LL_TkOvStChk_tiTrqChkT"
  Switch66/1 -> Bus Creator6/16  "LL_TkOvStChk_tiTDelTime"
  Data Type Conversion20/1 -> Switch55/2, Switch55/1
  Data Type Conversion77/1 -> Switch62/2, Switch62/1
  LLSMConClb31/1 -> Switch62/3
  Switch61/1 -> Bus Creator6/11  "LL_MAX_LONG_DECEL_DISABLE"
  LLSMConClb9/1 -> Switch88/3
  Switch73/1 -> Bus Creator6/8  "LL_MAX_DRIVER_TORQUE_DISABLE"
  Data Type Conversion10/1 -> Switch84/2, Switch84/1
  Data Type Conversion87/1 -> Switch75/1, Switch75/2
  LLSMConClb19/1 -> Switch59/3
  Switch78/1 -> Bus Creator7/7  "LL_DvtSpdDet_vDvtSpdMin_C"
  LLSMConClb26/1 -> Switch72/3
  Switch83/1 -> Bus Creator7/3  "LL_ThresDet_tiTTLCThresLDW"
  ICv to v10/1(Out1) -> Bus Creator6/2  "LL_MAX_LKAS_SPEED_DISABLE"
  LLSMConClb4/1 -> Switch58/3
  LLSMConClb16/1 -> Switch52/3
  LLSMConClb8/1 -> Switch87/3
  Switch77/1 -> Bus Creator7/6  "LL_ThresDet_tiTTLCThresLKA"
  ICv to v8/1(Out1) -> Bus Creator4/3  "LL_MIN_LKAS_SPEED_ENABLE"
  Switch74/1 -> Bus Creator6/9  "LL_MAX_STEER_SPEED_DISABLE"
  LLSMConClb24/1 -> Switch70/3
  LLSMConClb30/1 -> Switch61/3
  Switch80/1 -> ICv to v10/1(In1)
  ICv to v11/1(Out1) -> Bus Creator6/3  "LL_MIN_LKAS_SPEED_DISABLE"
  Bus Creator6/1 -> [DisblCClb]  "DisblCClb"
  Switch75/1 -> Bus Creator7/4  "LL_ThresDet_lDvtThresLwrLKA"
  Data Type Conversion44/1 -> Switch60/2, Switch60/1
  LLSMConClb21/1 -> Switch80/3
  LLSMConClb29/1 -> Switch79/3
  Switch63/1 -> Bus Creator6/13  "LL_MAX_DELAY_EPSSTAR_TIME"
  Data Type Conversion36/1 -> Switch52/2, Switch52/1
  Switch48/1 -> ICv to v7/1(In1)
  LLSMConClb7/1 -> Switch86/3
  Switch76/1 -> Bus Creator7/5  "LL_ThresDet_lDvtThresUprLKA"
  Switch51/1 -> Bus Creator4/15  "LL_DvtComp_C"
  Data Type Conversion19/1 -> Switch54/2, Switch54/1
  Data Type Conversion58/1 -> Switch80/2, Switch80/1
  Data Type Conversion82/1 -> Switch65/2, Switch65/1
  LLSMConClb18/1 -> Switch57/3
  Data Type Conversion72/1 -> Switch74/2, Switch74/1
  Switch79/1 -> Bus Creator6/10  "LL_MAX_LAT_ACC_DISABLE"
  Switch52/1 -> Bus Creator4/16  "LL_LDW_EarliestWarnLine_C"
  Data Type Conversion13/1 -> Switch81/2, Switch81/1
  Data Type Conversion88/1 -> Switch76/2, Switch76/1
  Switch64/1 -> Bus Creator6/14  "LL_Max_LDWS_Warning_Time"
  Data Type Conversion16/1 -> Switch49/2, Switch49/1
  LLSMConClb34/1 -> Switch65/3
  Switch70/1 -> Bus Creator6/5  "LL_MIN_LANE_WIDTH_DISABLE"
  Data Type Conversion84/1 -> Switch48/2, Switch48/1
  LLSMConClb27/1 -> Switch73/3
  Data Type Conversion11/1 -> Switch85/2, Switch85/1
  Switch53/1 -> Bus Creator4/11  "LL_MAX_LONG_DECEL_ENABLE"
  Data Type Conversion76/1 -> Switch61/1, Switch61/2
  Switch84/1 -> Bus Creator4/4  "LL_MAX_SYSTEM_CURVATURE_ENABLE"
  Data Type Conversion18/1 -> Switch53/2, Switch53/1
  Switch81/1 -> Bus Creator7/1  "LL_ThresDet_lDvtThresLwrLDW"
  LLSMConClb33/1 -> Switch64/3
  Data Type Conversion68/1 -> Switch72/2, Switch72/1
  Switch50/1 -> Bus Creator4/10  "LL_MAX_LAT_ACC_ENABLE"
  LLSMConClb40/1 -> Switch76/3
  Switch49/1 -> Bus Creator4/9  "LL_MAX_STEER_SPEED_ENABLE"
  LLSMConClb43/1 -> Switch49/3
  LLSMConClb25/1 -> Switch71/3
  Switch59/1 -> Bus Creator4/19  "LL_LKA_LatestWarnLine_C"
  LLSMConClb23/1 -> Switch68/3
  Switch85/1 -> Bus Creator4/5  "LL_MIN_LANE_WIDTH_ENABLE"
  Data Type Conversion70/1 -> Switch73/2, Switch73/1
  LLSMConClb37/1 -> Switch82/3
  LLSMConClb5/1 -> Switch84/3
  Data Type Conversion69/1 -> Switch67/2, Switch67/1
  LLSMConClb14/1 -> Switch56/3
  Data Type Conversion64/1 -> Switch70/2, Switch70/1
  LLSMConClb35/1 -> Switch66/3
  ICv to v7/1(Out1) -> Bus Creator4/2  "LL_MAX_LKAS_SPEED_ENABLE"
  Data Type Conversion14/1 -> Switch87/2, Switch87/1
  Data Type Conversion78/1 -> Switch63/2, Switch63/1
  Data Type Conversion17/1 -> Switch50/2, Switch50/1
  LLSMConClb38/1 -> Switch83/3
  Switch69/1 -> ICv to v11/1(In1)
  ICv to v9/1(Out1) -> Bus Creator6/1  "LL_MAX_LDWS_SPEED_DISABLE"
  Data Type Conversion65/1 -> Switch83/1, Switch83/2
  [LLL_MIN_LKAS_SPEED_DISABLE] -> Data Type Conversion67/1
  Bus Creator7/1 -> [ActvCClb]  "ActvCClb"
  Data Type Conversion46/1 -> Switch59/2, Switch59/1
  Switch82/1 -> Bus Creator7/2  "LL_ThresDet_lDvtThresUprLDW"
  Switch55/1 -> Bus Creator4/13  "LL_LKAS_OUT_OF_CONTROL_LAT_VEL"
  LLSMConClb12/1 -> Switch54/3
  LLSMConClb11/1 -> Switch53/3
  LLSMConClb39/1 -> Switch75/3
  Data Type Conversion66/1 -> Switch71/2, Switch71/1
  LLSMConClb41/1 -> Switch77/3
  LLSMConClb10/1 -> Switch50/3
  LLSMConClb3/1 -> Switch48/3
  ICv to v6/1(Out1) -> Bus Creator4/1  "LL_MAX_LDWS_SPEED_ENABLE"
  [EnaCClb] -> Bus Creator5/1
  [DisblCClb] -> Bus Creator5/2
  [ActvCClb] -> Bus Creator5/3
  Bus Creator5/1 -> LLSMConClb/1  "LLClb_bsLLSMConClb"
  Data Type Conversion22/1 -> Switch5/2, Switch5/1
  Switch5/1 -> Bus Creator4/20  "LL_LKA_EnableLine_Max"
  LLSMConClb1/1 -> Switch5/3
  LLSMConClb44/1 -> Switch6/3
  Data Type Conversion23/1 -> Switch6/2, Switch6/1
  Switch6/1 -> Bus Creator4/21  "LL_LKA_EnableLine_DvtMin"
  LLSMConClb45/1 -> Switch7/3
  Data Type Conversion24/1 -> Switch7/2, Switch7/1
  Switch7/1 -> Bus Creator4/22  "LL_LKA_EnableLine_DvtMax"

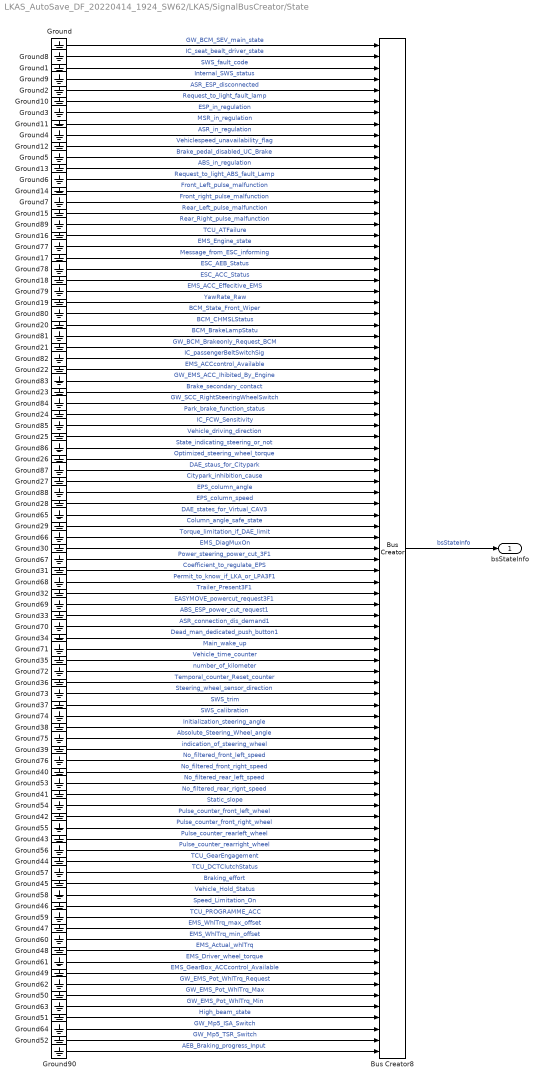
== system LKAS_AutoSave_DF_20220414_1924_SW62/LKAS/SignalBusCreator/State ==
  Bus Creator8 : BusCreator  Inputs=91
  Ground{,1..90} (91 alike) : Ground
  bsStateInfo : Outport
  wires:
  Ground1/1 -> Bus Creator8/3  "SWS_fault_code"
  Ground16/1 -> Bus Creator8/18  "TCU_ATFailure"
  Ground88/1 -> Bus Creator8/41  "EPS_column_angle"
  Ground62/1 -> Bus Creator8/85  "GW_EMS_Pot_WhlTrq_Request"
  Ground76/1 -> Bus Creator8/65  "No_filtered_front_left_speed"
  Ground61/1 -> Bus Creator8/83  "EMS_Driver_wheel_torque"
  Ground32/1 -> Bus Creator8/50  "Trailer_Present3F1"
  Ground34/1 -> Bus Creator8/54  "Dead_man_dedicated_push_button1"
  Ground35/1 -> Bus Creator8/56  "Vehicle_time_counter"
  Ground64/1 -> Bus Creator8/89  "GW_Mp5_ISA_Switch"
  Ground58/1 -> Bus Creator8/77  "Vehicle_Hold_Status"
  Ground81/1 -> Bus Creator8/27  "BCM_BrakeLampStatu"
  Ground82/1 -> Bus Creator8/29  "IC_passengerBeltSwitchSig"
  Ground78/1 -> Bus Creator8/21  "ESC_AEB_Status"
  Ground85/1 -> Bus Creator8/35  "IC_FCW_Sensitivity"
  Ground86/1 -> Bus Creator8/37  "State_indicating_steering_or_not"
  Ground87/1 -> Bus Creator8/39  "DAE_staus_for_Citypark"
  Ground49/1 -> Bus Creator8/84  "EMS_GearBox_ACCcontrol_Available"
  Ground48/1 -> Bus Creator8/82  "EMS_Actual_whlTrq"
  Ground45/1 -> Bus Creator8/76  "Braking_effort"
  Ground47/1 -> Bus Creator8/80  "EMS_WhlTrq_max_offset"
  Ground59/1 -> Bus Creator8/79  "TCU_PROGRAMME_ACC"
  Ground21/1 -> Bus Creator8/28  "GW_BCM_Brakeonly_Request_BCM"
  Ground56/1 -> Bus Creator8/73  "Pulse_counter_rearright_wheel"
  Ground2/1 -> Bus Creator8/5  "ASR_ESP_disconnected"
  Ground53/1 -> Bus Creator8/67  "No_filtered_rear_left_speed"
  Ground37/1 -> Bus Creator8/60  "SWS_trim"
  Ground4/1 -> Bus Creator8/9  "ASR_in_regulation"
  Ground74/1 -> Bus Creator8/61  "SWS_calibration"
  Ground70/1 -> Bus Creator8/53  "ASR_connection_dis_demand1"
  Ground68/1 -> Bus Creator8/49  "Permit_to_know_if_LKA_or_LPA3F1"
  Ground30/1 -> Bus Creator8/46  "EMS_DiagMuxOn"
  Ground29/1 -> Bus Creator8/44  "Column_angle_safe_state"
  Ground17/1 -> Bus Creator8/20  "Message_from_ESC_informing"
  Ground33/1 -> Bus Creator8/52  "ABS_ESP_power_cut_request1"
  Ground26/1 -> Bus Creator8/38  "Optimized_steering_wheel_torque"
  Ground84/1 -> Bus Creator8/33  "GW_SCC_RightSteeringWheelSwitch"
  Ground65/1 -> Bus Creator8/43  "DAE_states_for_Virtual_CAV3"
  Ground18/1 -> Bus Creator8/22  "ESC_ACC_Status"
  Ground27/1 -> Bus Creator8/40  "Citypark_inhibition_cause"
  Ground57/1 -> Bus Creator8/75  "TCU_DCTClutchStatus"
  Ground20/1 -> Bus Creator8/26  "BCM_CHMSLStatus"
  Ground39/1 -> Bus Creator8/64  "indication_of_steering_wheel"
  Ground69/1 -> Bus Creator8/51  "EASYMOVE_powercut_request3F1"
  Ground25/1 -> Bus Creator8/36  "Vehicle_driving_direction"
  Ground63/1 -> Bus Creator8/87  "GW_EMS_Pot_WhlTrq_Min"
  Ground54/1 -> Bus Creator8/69  "Static_slope"
  Ground52/1 -> Bus Creator8/90  "GW_Mp5_TSR_Switch"
  Ground73/1 -> Bus Creator8/59  "Steering_wheel_sensor_direction"
  Ground22/1 -> Bus Creator8/30  "EMS_ACCcontrol_Available"
  Ground89/1 -> Bus Creator8/17  "Rear_Right_pulse_malfunction"
  Ground31/1 -> Bus Creator8/48  "Coefficient_to_regulate_EPS"
  Ground9/1 -> Bus Creator8/4  "Internal_SWS_status"
  Ground72/1 -> Bus Creator8/57  "number_of_kilometer"
  Ground66/1 -> Bus Creator8/45  "Torque_limitation_if_DAE_limit"
  Ground6/1 -> Bus Creator8/13  "Request_to_light_ABS_fault_Lamp"
  Ground24/1 -> Bus Creator8/34  "Park_brake_function_status"
  Ground15/1 -> Bus Creator8/16  "Rear_Left_pulse_malfunction"
  Ground60/1 -> Bus Creator8/81  "EMS_WhlTrq_min_offset"
  Ground23/1 -> Bus Creator8/32  "Brake_secondary_contact"
  Ground5/1 -> Bus Creator8/11  "Brake_pedal_disabled_UC_Brake"
  Ground13/1 -> Bus Creator8/12  "ABS_in_regulation"
  Ground10/1 -> Bus Creator8/6  "Request_to_light_fault_lamp"
  Ground50/1 -> Bus Creator8/86  "GW_EMS_Pot_WhlTrq_Max"
  Ground11/1 -> Bus Creator8/8  "MSR_in_regulation"
  Ground36/1 -> Bus Creator8/58  "Temporal_counter_Reset_counter"
  Ground3/1 -> Bus Creator8/7  "ESP_in_regulation"
  Ground40/1 -> Bus Creator8/66  "No_filtered_front_right_speed"
  Ground51/1 -> Bus Creator8/88  "High_beam_state"
  Ground46/1 -> Bus Creator8/78  "Speed_Limitation_On"
  Ground83/1 -> Bus Creator8/31  "GW_EMS_ACC_Ihibited_By_Engine"
  Ground19/1 -> Bus Creator8/24  "YawRate_Raw"
  Ground38/1 -> Bus Creator8/62  "Initialization_steering_angle"
  Ground90/1 -> Bus Creator8/91  "AEB_Braking_progress_Input"
  Bus Creator8/1 -> bsStateInfo/1  "bsStateInfo"
  Ground67/1 -> Bus Creator8/47  "Power_steering_power_cut_3F1"
  Ground41/1 -> Bus Creator8/68  "No_filtered_rear_rignt_speed"
  Ground80/1 -> Bus Creator8/25  "BCM_State_Front_Wiper"
  Ground77/1 -> Bus Creator8/19  "EMS_Engine_state"
  Ground79/1 -> Bus Creator8/23  "EMS_ACC_Effecitive_EMS"
  Ground28/1 -> Bus Creator8/42  "EPS_column_speed"
  Ground7/1 -> Bus Creator8/15  "Front_right_pulse_malfunction"
  Ground55/1 -> Bus Creator8/71  "Pulse_counter_front_right_wheel"
  Ground44/1 -> Bus Creator8/74  "TCU_GearEngagement"
  Ground71/1 -> Bus Creator8/55  "Main_wake_up"
  Ground75/1 -> Bus Creator8/63  "Absolute_Steering_Wheel_angle"
  Ground12/1 -> Bus Creator8/10  "Vehiclespeed_unavailability_flag"
  Ground43/1 -> Bus Creator8/72  "Pulse_counter_rearleft_wheel"
  Ground42/1 -> Bus Creator8/70  "Pulse_counter_front_left_wheel"
  Ground/1 -> Bus Creator8/1  "GW_BCM_SEV_main_state"
  Ground8/1 -> Bus Creator8/2  "IC_seat_bealt_driver_state"
  Ground14/1 -> Bus Creator8/14  "Front_Left_pulse_malfunction"
